simulink model "Brakes_wStatic"  (R2020a)
settings: Solver=VariableStepAuto  StartTime=0.0  StopTime=10.0  RelTol=1e-3
undefined symbols (not defined in the file): Brake_bias, Brake_radius, Effective_radius
settings Model: DataDictionary=Properties.sldd  Creator=Matthew  LastModifiedBy=Matthew

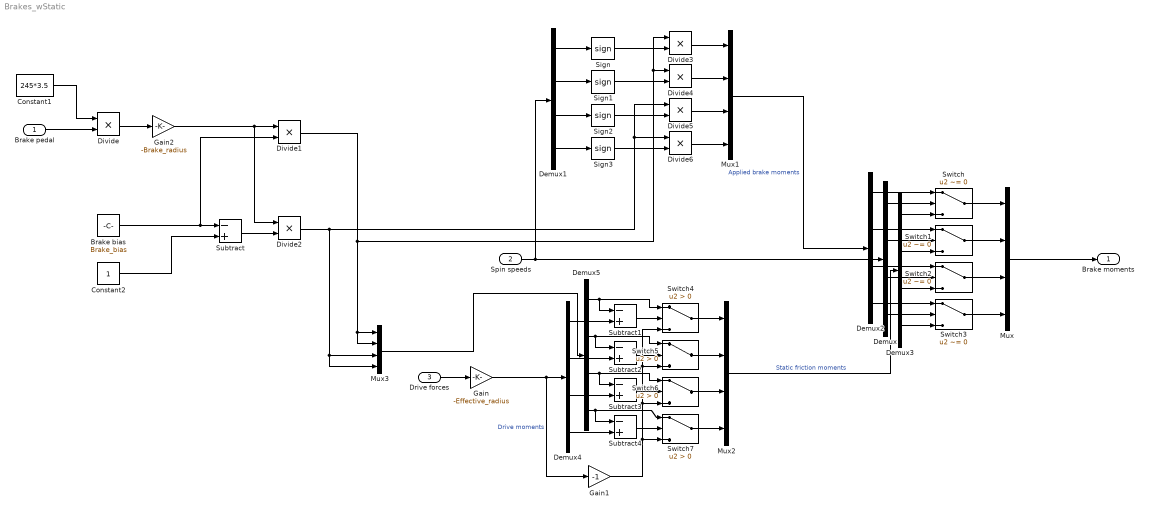
== system Brakes_wStatic ==
  Brake pedal : Inport
  Spin speeds : Inport  Port=2
  Drive forces : Inport  Port=3
  Brake bias : Constant  Value=Brake_bias
  Constant1 : Constant  Value=245*3.5
  Constant2 : Constant
  Demux{,1..5} (6 alike) : Demux
  Divide{,1..6} (7 alike) : Product  Inputs=**
  Gain : Gain  Gain=-Effective_radius
  Gain1 : Gain  Gain=-1
  Gain2 : Gain  Gain=-Brake_radius
  Mux{,1..3} (4 alike) : Mux
  Sign{,1..3} (4 alike) : Signum
  Subtract{,1..4} (5 alike) : Sum  Inputs=-+
  Switch{,1..3} (4 alike) : Switch  Criteria=u2 ~= 0
  Switch{4..7} (4 alike) : Switch  Criteria=u2 > Threshold
  Brake moments : Outport
  wires:
  Brake pedal/1 -> Divide/2
  Constant1/1 -> Divide/1
  Divide/1 -> Gain2/1
  Brake bias/1 -> Subtract/1, Divide1/2
  Divide1/1 -> Divide3/1, Divide4/1, Mux3/2, Mux3/1
  Constant2/1 -> Subtract/2
  Divide2/1 -> Divide5/1, Divide6/1, Mux3/4, Mux3/3
  Subtract/1 -> Divide2/2
  Spin speeds/1 -> Demux1/1, Demux/1
  Demux/1 -> Switch/2
  Demux/2 -> Switch1/2
  Demux/3 -> Switch2/2
  Demux/4 -> Switch3/2
  Drive forces/1 -> Gain/1
  Switch/1 -> Mux/1
  Switch1/1 -> Mux/2
  Switch2/1 -> Mux/3
  Switch3/1 -> Mux/4
  Mux/1 -> Brake moments/1
  Divide3/1 -> Mux1/1
  Sign/1 -> Divide3/2
  Demux1/1 -> Sign/1
  Demux1/2 -> Sign1/1
  Demux1/3 -> Sign2/1
  Demux1/4 -> Sign3/1
  Sign1/1 -> Divide4/2
  Sign2/1 -> Divide5/2
  Sign3/1 -> Divide6/2
  Divide4/1 -> Mux1/2
  Divide5/1 -> Mux1/3
  Divide6/1 -> Mux1/4
  Demux2/1 -> Switch/1
  Demux2/2 -> Switch1/1
  Demux2/3 -> Switch2/1
  Demux2/4 -> Switch3/1
  Mux1/1 -> Demux2/1  "Applied brake moments"
  Demux3/1 -> Switch/3
  Demux3/2 -> Switch1/3
  Demux3/3 -> Switch2/3
  Demux3/4 -> Switch3/3
  Mux2/1 -> Demux3/1  "Static friction moments"
  Gain/1 -> Gain1/1, Demux4/1  "Drive moments"
  Demux5/1 -> Switch4/1, Subtract1/1
  Demux4/1 -> Subtract1/2
  Demux5/2 -> Switch5/1, Subtract2/1
  Demux5/4 -> Switch7/1, Subtract4/1
  Demux5/3 -> Switch6/1, Subtract3/1
  Demux4/2 -> Subtract2/2
  Demux4/3 -> Subtract3/2
  Demux4/4 -> Subtract4/2
  Subtract1/1 -> Switch4/2
  Subtract2/1 -> Switch5/2
  Subtract3/1 -> Switch6/2
  Subtract4/1 -> Switch7/2
  Gain1/1 -> Switch7/3, Switch6/3, Switch4/3, Switch5/3
  Switch4/1 -> Mux2/1
  Switch5/1 -> Mux2/2
  Switch6/1 -> Mux2/3
  Switch7/1 -> Mux2/4
  Mux3/1 -> Demux5/1
  Gain2/1 -> Divide1/1, Divide2/1
